simulink model "sampleModel33"  (R2021b)
settings: Solver=VariableStepAuto  StartTime=0.0  StopTime=10.0  RelTol=1e-3
undefined symbols (not defined in the file or in its folder): DiscIntNeverNeededParam, Newton, Raphson
libraries: simulink x17, slpidlib x2
settings Model: Creator=user  LastModifiedBy=user

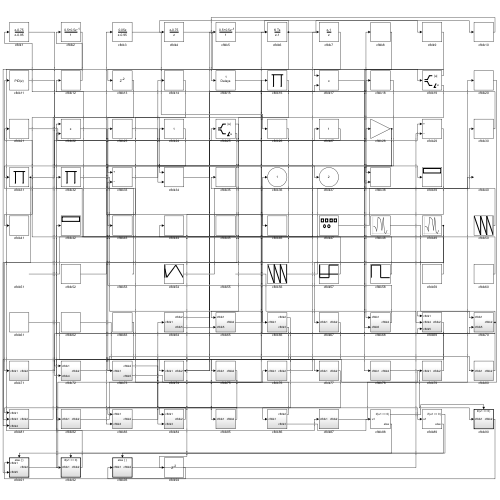
[thumbnail: Simulink's stored preview of the top-level diagram]
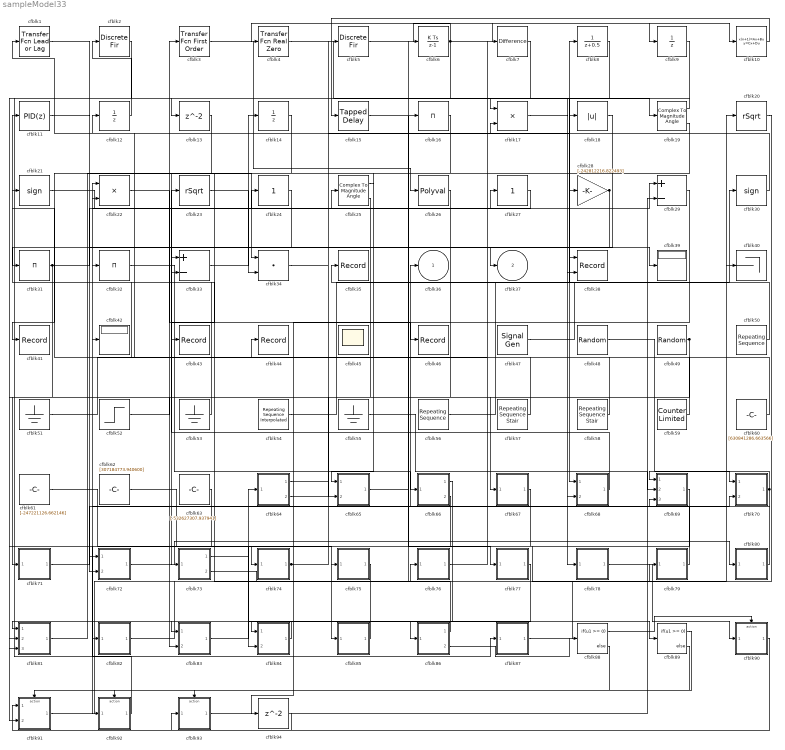
== system sampleModel33 ==
  cfblk1 : simulink/Discrete/Transfer Fcn Lead or Lag  PoleZ=0.95  ZeroZ=0.75  ICPrevOutput=0.0  ICPrevInput=0.0  DoSatur=off
      settings: SourceProductBaseCode=SL
  cfblk10 : DiscreteStateSpace
  cfblk11 : slpidlib/PID Controller  Controller=PID  Form=Parallel  TimeDomain=Discrete-time  UseExternalTs=off  SampleTime=1  IntegratorMethod=Forward Euler  FilterMethod=Forward Euler  ControllerParametersSource=internal  P=1  I=1  D=0  UseFilter=on  N=100  TunerSelectOption=Transfer Function Based (PID Tuner App)  InitialConditionSource=internal  InitialConditionForIntegrator=0  InitialConditionForFilter=0  DifferentiatorICPrevScaledInput=0  ExternalReset=none  TrackingMode=off  Kt=1  LimitOutput=off  SatLimitsSource=internal  UpperSaturationLimit=inf  LowerSaturationLimit=-inf  LinearizeAsGain=off  AntiWindupMode=none  Kb=1  POutMin=[]  POutMax=[]  IOutMin=[]  IOutMax=[]  DOutMin=[]  DOutMax=[]  NOutMin=[]  NOutMax=[]  SumOutMin=[]  SumOutMax=[]  SaturationOutMin=[]  SaturationOutMax=[]  PParamMin=[]  PParamMax=[]  IParamMin=[]  IParamMax=[]  DParamMin=[]  DParamMax=[]  NParamMin=[]  NParamMax=[]  KbParamMin=[]  KbParamMax=[]  KtParamMin=[]  KtParamMax=[]  KbOutMin=[]  KbOutMax=[]  KtOutMin=[]  KtOutMax=[]  IntegratorOutMin=[]  IntegratorOutMax=[]  FilterOutMin=[]  FilterOutMax=[]  SumI1OutMin=[]  SumI1OutMax=[]  SumI2OutMin=[]  SumI2OutMax=[]  SumI3OutMin=[]  SumI3OutMax=[]  SumI4OutMin=[]  SumI4OutMax=[]  SumDOutMin=[]  SumDOutMax=[]  DifferentiatorOutMin=[]  DifferentiatorOutMax=[]  FilterDiffOutCoefMin=[]  FilterDiffOutCoefMax=[]  ReciprocalOutMin=[]  ReciprocalOutMax=[]  SumDenOutMin=[]  SumDenOutMax=[]  SumNumOutMin=[]  SumNumOutMax=[]  DivideOutMin=[]  DivideOutMax=[]  UdiffTsProdOutMin=[]  UdiffTsProdOutMax=[]  NTsProdOutMin=[]  NTsProdOutMax=[]  UintegralTsProdOutMin=[]  UintegralTsProdOutMax=[]  UngainTsProdOutMin=[]  UngainTsProdOutMax=[]  IntegratorContinuousStateAttributes=''  IntegratorStateMustResolveToSignalObject=off  IntegratorRTWStateStorageClass=Auto  FilterContinuousStateAttributes=''  FilterStateMustResolveToSignalObject=off  FilterRTWStateStorageClass=Auto  ParallelPVariant=InternalParameters  IdealPVariant=Disabled  IVariant=InternalParameters  DVariant=InternalParameters  IntegratorVariant=Discrete  SatVariant=Disabled  AWVariant=Passthrough  PCopyVariant=Disabled  TRVariant=Disabled  FdbkBlocksVariant=Forward  IdealPFdbkVariant=Disabled  SatFdbkVariant=Disabled  DerivativeFilterVariant=ForwardEulerFilter  NVariant=InternalParameters  NCopyVariant=Disabled  FilterICVariant=InternalICsFilter  IntegratorICVariant=InternalICs  ExternalResetVariant=Disabled  TRSumVariant=Passthrough  SumFdbkVariant=Disabled  SumVariant=Sum_PID  TsampFilterVariant=InternalTs  TsampNgainVariant=Passthrough  TsampIntegralVariant=Passthrough  ExternalSaturationOutDataTypeStr=Inherit: Same as second input
  cfblk12 : UnitDelay  HasFrameUpgradeWarning=on
  cfblk13 : Delay  SampleTime=1
  cfblk14 : UnitDelay  HasFrameUpgradeWarning=on
  cfblk15 : simulink/Discrete/Tapped Delay  vinit=0.0  samptime=-1  NumDelays=1  DelayOrder=Oldest  includeCurrent=off
  cfblk16 : Product  Inputs=*
  cfblk17 : Product
  cfblk18 : Abs
  cfblk19 : ComplexToMagnitudeAngle
  cfblk2 : DiscreteFir  SampleTime=1
  cfblk20 : Sqrt  Operator=rSqrt  AlgorithmType=Newton-Raphson  SaturateOnIntegerOverflow=on
  cfblk21 : Signum
  cfblk22 : Product
  cfblk23 : Sqrt  Operator=rSqrt  AlgorithmType=Newton-Raphson  SaturateOnIntegerOverflow=on
  cfblk24 : simulink/Math Operations/Slider Gain  gain=1  low=0  high=2
  cfblk25 : ComplexToMagnitudeAngle
  cfblk26 : Polyval  Coefs=[ +2.081618890e-019, -1.441693666e-014, +4.719686976e-010, -8.536869453e-006, +1.621573104e-001, -8.087801117e+001 ]
  cfblk27 : simulink/Math Operations/Slider Gain  gain=1  low=0  high=2
  cfblk28 : Gain  Gain=[-242812216.822493]
  cfblk29 : Sum  Inputs=+-
  cfblk3 : simulink/Discrete/Transfer Fcn First Order  PoleZ=0.95  ICPrevOutput=0.0  DoSatur=off
  cfblk30 : Signum
  cfblk31 : Product  Inputs=*
  cfblk32 : Product  Inputs=*
  cfblk33 : Sum  Inputs=+-
  cfblk34 : DotProduct  InputSameDT=on  OutDataTypeStr=Inherit: Inherit via internal rule
  cfblk35 : Record  FileSettingsInternal="{\"entries\":[{\"content\":{\"excelSettings\":{\"content\":{},\"type\":\"Streamout.ExcelSettings\"}},\"type\":\"Streamout.FileSettingStorage\",\"uuid\":\"35001ed6-113c-4df0-b2ca-dfb1ae9641fd\"}],\"packageUris\":[\"http://schema.mathworks.com/mf0/streamout_blocks/R2020a\"],\"version\":\"1.0\"}"  SignalsInternal="{\"entries\":[{\"content\":{\"signals\":[{\"content\":{\"blockPath\":[\"sampleModel33/cfblk35\"],\"channel\":[],\"dimensions\":[1],\"domain\":\"sampleModel33/cfblk35\",\"lineColor\":\"#7e2f8e\",\"plots\":[1],\"port\":1,\"sid\":[\"\"],\"signalID\":1315,\"signalName\":\"cfblk50\"},\"type\":\"RecordBlkView.Signal\",\"uuid\":\"b51956be-35d7-410c-a634-2c74a70fc2db\"}]},\"type\":\"RecordBlkView.InputSignals\",\"uuid\":\"6f3c5769-0a70-4b4d-8f9e-08021210cbdc\"}],\"packageUris\":[\"http://schema.mathworks.com/mf0/streamout_blocks/R2020a\"],\"version\":\"1.0\"}"  VisualizationBindings="{\"sparklinesplugin\":{\"info\":[{\"bindingParametersList\":[],\"subplotID\":1}]}}"
  cfblk38 : Record  FileSettingsInternal="{\"entries\":[{\"content\":{\"excelSettings\":{\"content\":{},\"type\":\"Streamout.ExcelSettings\"}},\"type\":\"Streamout.FileSettingStorage\",\"uuid\":\"0be8a96a-0af5-42bf-ad20-4a59eb5ad2b5\"}],\"packageUris\":[\"http://schema.mathworks.com/mf0/streamout_blocks/R2020a\"],\"version\":\"1.0\"}"  Layout=[1 1]  SignalsInternal="{\"entries\":[{\"content\":{\"signals\":[{\"content\":{\"blockPath\":[\"sampleModel33/cfblk38\"],\"channel\":[],\"dimensions\":[1],\"domain\":\"sampleModel33/cfblk38\",\"lineColor\":\"#a2142f\",\"plots\":[1],\"port\":1,\"sid\":[\"\"],\"signalID\":1291,\"signalName\":\"cfblk18\"},\"type\":\"RecordBlkView.Signal\",\"uuid\":\"6335e883-a2f0-4c07-b781-486b19723835\"},{\"content\":{\"blockPath\":[\"sampleModel33/cfblk38\"],\"channel\":[],\"dimensions\":[1],\"domain\":\"sampleModel33/cfblk38\",\"lineColor\":\"#139fff\",\"plots\":[1],\"port\":2,\"sid\":[\"\"],\"signalID\":1295,\"signalName\":\"cfblk28\"},\"type\":\"RecordBlkView.Signal\",\"uuid\":\"6659cc2e-0a72-45a6-80d2-b962cd38ef36\"}]},\"type\":\"RecordBlkView.InputSignals\",\"uuid\":\"964d8c4e-428f-4cc5-8505-fdd76ce85f40\"}],\"packageUris\":[\"http://schema.mathworks.com/mf0/streamout_blocks/R2020a\"],\"version\":\"1.0\"}"  VisualizationBindings="{\"xyplotplugin\":{\"info\":[{\"series\":[{\"bindingParametersList\":[{\"parameter\":\"X-Axis\",\"signalID\":1291,\"signalName\":\"cfblk18\"},{\"parameter\":\"Y-Axis\",\"signalID\":1295,\"signalName\":\"cfblk28\"}],\"seriesID\":40894}],\"subplotID\":1}]}}"  CompatibilityTag=XY
  cfblk39 : Display
  cfblk4 : simulink/Discrete/Transfer Fcn Real Zero  ZeroZ=0.75  ICPrevInput=0.0  DoSatur=off
      settings: SourceProductBaseCode=SL
  cfblk40 : Terminator
  cfblk41 : Record  FileSettingsInternal="{\"entries\":[{\"content\":{\"excelSettings\":{\"content\":{},\"type\":\"Streamout.ExcelSettings\"}},\"type\":\"Streamout.FileSettingStorage\",\"uuid\":\"943cf604-ea0c-4e86-a751-38b2b14ebefe\"}],\"packageUris\":[\"http://schema.mathworks.com/mf0/streamout_blocks/R2020a\"],\"version\":\"1.0\"}"  SignalsInternal="{\"entries\":[{\"content\":{\"signals\":[{\"content\":{\"blockPath\":[\"sampleModel33/cfblk41\"],\"channel\":[],\"dimensions\":[1],\"domain\":\"sampleModel33/cfblk41\",\"lineColor\":\"#22b573\",\"plots\":[1],\"port\":1,\"sid\":[\"\"],\"signalID\":1299,\"signalName\":\"cfblk14\"},\"type\":\"RecordBlkView.Signal\",\"uuid\":\"e871c3d6-6255-463e-9a74-0a0ab0dc3673\"}]},\"type\":\"RecordBlkView.InputSignals\",\"uuid\":\"e3ee7eed-40cd-48d9-8ee8-8000d3adafc3\"}],\"packageUris\":[\"http://schema.mathworks.com/mf0/streamout_blocks/R2020a\"],\"version\":\"1.0\"}"  VisualizationBindings="{\"sparklinesplugin\":{\"info\":[{\"bindingParametersList\":[],\"subplotID\":1}]}}"
  cfblk42 : Display
  cfblk43 : Record  FileSettingsInternal="{\"entries\":[{\"content\":{\"excelSettings\":{\"content\":{},\"type\":\"Streamout.ExcelSettings\"}},\"type\":\"Streamout.FileSettingStorage\",\"uuid\":\"3f9b25bd-badb-4d41-b468-b463b58841fb\"}],\"packageUris\":[\"http://schema.mathworks.com/mf0/streamout_blocks/R2020a\"],\"version\":\"1.0\"}"  SignalsInternal="{\"entries\":[{\"content\":{\"signals\":[{\"content\":{\"blockPath\":[\"sampleModel33/cfblk43\"],\"channel\":[],\"dimensions\":[1],\"domain\":\"sampleModel33/cfblk43\",\"lineColor\":\"#0072bd\",\"plots\":[1],\"port\":1,\"sid\":[\"\"],\"signalID\":1303,\"signalName\":\"cfblk19:2\"},\"type\":\"RecordBlkView.Signal\",\"uuid\":\"9792fccf-e420-4e25-ab06-4eadf706866a\"}]},\"type\":\"RecordBlkView.InputSignals\",\"uuid\":\"96c16f90-f0aa-40b6-afa4-1459bd73ce77\"}],\"packageUris\":[\"http://schema.mathworks.com/mf0/streamout_blocks/R2020a\"],\"version\":\"1.0\"}"  VisualizationBindings="{\"sparklinesplugin\":{\"info\":[{\"bindingParametersList\":[],\"subplotID\":1}]}}"
  cfblk44 : Record  FileSettingsInternal="{\"entries\":[{\"content\":{\"excelSettings\":{\"content\":{},\"type\":\"Streamout.ExcelSettings\"}},\"type\":\"Streamout.FileSettingStorage\",\"uuid\":\"f2588ed7-79e1-4caa-a079-da7ab20d12fc\"}],\"packageUris\":[\"http://schema.mathworks.com/mf0/streamout_blocks/R2020a\"],\"version\":\"1.0\"}"  SignalsInternal="{\"entries\":[{\"content\":{\"signals\":[{\"content\":{\"blockPath\":[\"sampleModel33/cfblk44\"],\"channel\":[],\"dimensions\":[1],\"domain\":\"sampleModel33/cfblk44\",\"lineColor\":\"#77ac30\",\"plots\":[1],\"port\":1,\"sid\":[\"\"],\"signalID\":1319,\"signalName\":\"cfblk58\"},\"type\":\"RecordBlkView.Signal\",\"uuid\":\"acc73365-e21f-4d8b-96ab-155052806760\"}]},\"type\":\"RecordBlkView.InputSignals\",\"uuid\":\"d7a8ec08-6dc6-46d4-b733-eb162bbe280f\"}],\"packageUris\":[\"http://schema.mathworks.com/mf0/streamout_blocks/R2020a\"],\"version\":\"1.0\"}"  VisualizationBindings="{\"sparklinesplugin\":{\"info\":[{\"bindingParametersList\":[],\"subplotID\":1}]}}"
  cfblk45 : Scope
      settings: Floating=on
  cfblk46 : Record  FileSettingsInternal="{\"entries\":[{\"content\":{\"excelSettings\":{\"content\":{},\"type\":\"Streamout.ExcelSettings\"}},\"type\":\"Streamout.FileSettingStorage\",\"uuid\":\"2d09eccc-ab10-47b1-af95-cecebc9448e0\"}],\"packageUris\":[\"http://schema.mathworks.com/mf0/streamout_blocks/R2020a\"],\"version\":\"1.0\"}"  SignalsInternal="{\"entries\":[{\"content\":{\"signals\":[{\"content\":{\"blockPath\":[\"sampleModel33/cfblk46\"],\"channel\":[],\"dimensions\":[1],\"domain\":\"sampleModel33/cfblk46\",\"lineColor\":\"#d95319\",\"plots\":[1],\"port\":1,\"sid\":[\"\"],\"signalID\":1307,\"signalName\":\"cfblk22\"},\"type\":\"RecordBlkView.Signal\",\"uuid\":\"5f2a2cab-08a1-4387-b816-50fa2120540d\"}]},\"type\":\"RecordBlkView.InputSignals\",\"uuid\":\"c9b5cd79-e6b9-468f-9bb4-0740aaf235d3\"}],\"packageUris\":[\"http://schema.mathworks.com/mf0/streamout_blocks/R2020a\"],\"version\":\"1.0\"}"  VisualizationBindings="{\"sparklinesplugin\":{\"info\":[{\"bindingParametersList\":[],\"subplotID\":1}]}}"
  cfblk47 : SignalGenerator  WaveForm=sawtooth  Amplitude=[-806395238.078433]
  cfblk48 : RandomNumber  Mean=[46041.065691]  Variance=[79471.340689]  Seed=[573569622.000000]  SampleTime=0.1
  cfblk49 : RandomNumber  Mean=[-27661.970417]  Variance=[16133.365811]  Seed=[886370585.000000]  SampleTime=0.1
  cfblk5 : DiscreteFir  SampleTime=1
  cfblk50 : simulink/Sources/Repeating Sequence  rep_seq_t=[0 2]  rep_seq_y=[803997380.811525, 517164280.997497]
  cfblk51 : Ground
  cfblk52 : Step  Time=[18.000000]  Before=[-7550237.569274]  After=[317370971.728037]  SampleTime=0
  cfblk53 : Ground
  cfblk54 : simulink/Sources/Repeating Sequence Interpolated  OutValues=[-422066434.065173, -713885697.695092, -383733753.736717, -305117400.776015, -720923073.966345]  TimeValues=[0 0.1 0.5 0.6 1].'  LookUpMeth=Interpolation-Use End Values  tsamp=0.01  OutMin=[]  OutMax=[]  OutDataTypeStr=double  OutputDataTypeScalingMode=double  OutDataType=fixdt(0,8)  OutScaling=2^-10
  cfblk55 : Ground
  cfblk56 : simulink/Sources/Repeating Sequence  rep_seq_t=[0 2]  rep_seq_y=[111643374.462294, -897632520.777855]
  cfblk57 : simulink/Sources/Repeating Sequence Stair  OutValues=[-165294741.865797, 423160325.966491]  tsamp=-1  OutMin=[]  OutMax=[]  OutDataTypeStr=double  OutputDataTypeScalingMode=double  OutDataType=fixdt(0,8)  ConRadixGroup=Best Precision: Vector-wise  OutScaling=2^-12
  cfblk58 : simulink/Sources/Repeating Sequence Stair  OutValues=[758546070.290987, 202958879.064606]  tsamp=-1  OutMin=[]  OutMax=[]  OutDataTypeStr=double  OutputDataTypeScalingMode=double  OutDataType=fixdt(0,8)  ConRadixGroup=Best Precision: Vector-wise  OutScaling=2^-12
  cfblk59 : simulink/Sources/Counter Limited  uplimit=[465.000000]  tsamp=-1
  cfblk6 : DiscreteIntegrator  ICPrevOutput=DiscIntNeverNeededParam  ICPrevScaledInput=DiscIntNeverNeededParam
  cfblk60 : Constant  Value=[630841286.663566]  SampleTime=1
  cfblk61 : Constant  Value=[-247221126.662146]  SampleTime=1
  cfblk62 : Constant  Value=[307184773.940600]  SampleTime=1
  cfblk63 : Constant  Value=[-532627307.937941]  SampleTime=1
  cfblk64 : Subsystem
  cfblk65 : Subsystem
  cfblk66 : Subsystem
  cfblk67 : Subsystem
  cfblk68 : Subsystem
  cfblk69 : Subsystem
  cfblk7 : simulink/Discrete/Difference  ICPrevInput=0.0  OutMin=[]  OutMax=[]  OutDataTypeStr=Inherit: Inherit via back propagation  OutDataType=fixdt(1, 16)  OutScaling=2^-10  DoSatur=off
  cfblk70 : Subsystem
  cfblk71 : Subsystem
  cfblk72 : Subsystem
  cfblk73 : Subsystem
  cfblk74 : Subsystem
  cfblk75 : Subsystem
  cfblk76 : Subsystem
  cfblk77 : Subsystem
  cfblk78 : Subsystem
  cfblk79 : Subsystem
  cfblk8 : DiscreteTransferFcn  SampleTime=1
  cfblk80 : Subsystem
  cfblk81 : Subsystem
  cfblk82 : Subsystem
  cfblk83 : Subsystem
  cfblk84 : Subsystem
  cfblk85 : Subsystem
  cfblk86 : Subsystem
  cfblk87 : Subsystem
  cfblk88 : If  IfExpression=u1 >= 0  SampleTime=1
  cfblk89 : If  IfExpression=u1 >= 0  SampleTime=1
  cfblk9 : UnitDelay  HasFrameUpgradeWarning=on
  cfblk90 : Subsystem  TreatAsAtomicUnit=on
  cfblk91 : Subsystem  TreatAsAtomicUnit=on
  cfblk92 : Subsystem  TreatAsAtomicUnit=on
  cfblk93 : Subsystem  TreatAsAtomicUnit=on
  cfblk94 : Delay  SampleTime=1
  cfblk36 : Outport
  cfblk37 : Outport  Port=2
  wires:
  cfblk80/1(cfblk2) -> cfblk22/1
  cfblk77/1(cfblk2) -> cfblk86/1(cfblk1)
  cfblk20/1 -> cfblk74/1(cfblk1)
  cfblk78/1(cfblk2) -> cfblk90/1(cfblk1)
  cfblk72/1(cfblk2) -> cfblk80/1(cfblk1)
  cfblk81/1(cfblk2) -> cfblk34/1
  cfblk2/1 -> cfblk87/1(cfblk1)
  cfblk48/1 -> cfblk70/1(cfblk1)
  cfblk92/1(cfblk2) -> cfblk42/1
  cfblk91/1(cfblk2) -> cfblk79/1(cfblk1)
  cfblk21/1 -> cfblk24/1
  cfblk27/1 -> cfblk22/2
  cfblk23/1 -> cfblk39/1
  cfblk62/1 -> cfblk85/1(cfblk1)
  cfblk13/1 -> cfblk73/1(cfblk1)
  cfblk5/1 -> cfblk9/1
  cfblk58/1 -> cfblk44/1
  cfblk3/1 -> cfblk26/1
  cfblk53/1 -> cfblk11/1
  cfblk69/1(cfblk2) -> cfblk75/1(cfblk1)
  cfblk73/1(cfblk2) -> cfblk89/1
  cfblk28/1 -> cfblk31/1, cfblk38/2
  cfblk56/1 -> cfblk8/1
  cfblk10/1 -> cfblk15/1
  cfblk49/1 -> cfblk71/1(cfblk1), cfblk67/1(cfblk1)
  cfblk9/1 -> cfblk68/1(cfblk1)
  cfblk59/1 -> cfblk32/1
  cfblk85/1(cfblk2) -> cfblk81/1(cfblk1)
  cfblk31/1 -> cfblk25/1, cfblk81/3(cfblk4)
  cfblk65/1(cfblk2) -> cfblk6/1
  cfblk82/1(cfblk2) -> cfblk16/1
  cfblk47/1 -> cfblk30/1
  cfblk7/1 -> cfblk13/1
  cfblk73/2(cfblk5) -> cfblk76/1(cfblk1)
  cfblk79/1(cfblk2) -> cfblk36/1
  cfblk16/1 -> cfblk65/1(cfblk1)
  cfblk12/1 -> cfblk2/1
  cfblk68/1(cfblk2) -> cfblk23/1
  cfblk15/1 -> cfblk77/1(cfblk1)
  cfblk17/1 -> cfblk78/1(cfblk1)
  cfblk8/1 -> cfblk68/2(cfblk5)
  cfblk76/1(cfblk2) -> cfblk29/1
  cfblk87/1(cfblk2) -> cfblk40/1
  cfblk57/1 -> cfblk21/1
  cfblk33/1 -> cfblk14/1
  cfblk66/1(cfblk2) -> cfblk84/1(cfblk1)
  cfblk52/1 -> cfblk3/1
  cfblk32/1 -> cfblk66/1(cfblk1)
  cfblk60/1 -> cfblk12/1
  cfblk90/1(cfblk2) -> cfblk91/1(cfblk1)
  cfblk75/1(cfblk2) -> cfblk92/1(cfblk1)
  cfblk83/1(cfblk2) -> cfblk64/1(cfblk1)
  cfblk67/1(cfblk2) -> cfblk82/1(cfblk1)
  cfblk6/1 -> cfblk10/1, cfblk4/1, cfblk91/2(cfblk5)
  cfblk11/1 -> cfblk37/1
  cfblk25/1 -> cfblk34/2
  cfblk93/1(cfblk2) -> cfblk29/2
  cfblk84/1(cfblk2) -> cfblk83/1(cfblk1)
  cfblk4/1 -> cfblk19/1
  cfblk63/1 -> cfblk81/2(cfblk3)
  cfblk22/1 -> cfblk46/1
  cfblk14/1 -> cfblk41/1
  cfblk24/1 -> cfblk33/1
  cfblk74/1(cfblk2) -> cfblk27/1, cfblk17/2
  cfblk26/1 -> cfblk83/2(cfblk3)
  cfblk64/1(cfblk2) -> cfblk28/1
  cfblk1/1 -> cfblk72/1(cfblk1)
  cfblk19/1 -> cfblk17/1
  cfblk71/1(cfblk2) -> cfblk70/2(cfblk5)
  cfblk64/2(cfblk5) -> cfblk18/1
  cfblk34/1 -> cfblk5/1
  cfblk61/1 -> cfblk84/2(cfblk3)
  cfblk70/1(cfblk2) -> cfblk69/1(cfblk1), cfblk69/3(cfblk5)
  cfblk54/1 -> cfblk20/1
  cfblk86/1(cfblk2) -> cfblk33/2
  cfblk66/2(cfblk3) -> cfblk72/2(cfblk4)
  cfblk55/1 -> cfblk69/2(cfblk4)
  cfblk18/1 -> cfblk38/1
  cfblk51/1 -> cfblk7/1
  cfblk30/1 -> cfblk1/1
  cfblk86/2(cfblk3) -> cfblk88/1
  cfblk19/2 -> cfblk43/1
  cfblk25/2 -> cfblk65/2(cfblk5)
  cfblk50/1 -> cfblk35/1
  cfblk88/1 -> cfblk90/Action
  cfblk88/2 -> cfblk91/Action
  cfblk89/1 -> cfblk92/Action
  cfblk89/2 -> cfblk93/Action
  cfblk29/1 -> cfblk94/1
  cfblk94/1 -> cfblk93/1(cfblk1)

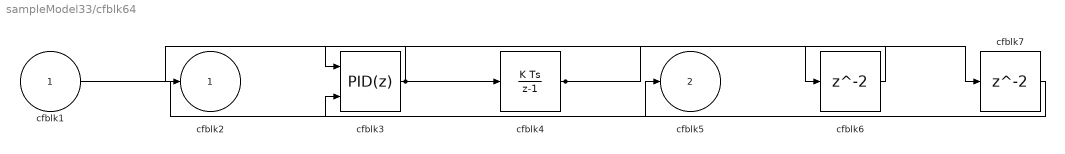
== system sampleModel33/cfblk64 ==
  cfblk1 : Inport
  cfblk3 : slpidlib/PID Controller (2DOF)  Controller=PID  Form=Parallel  TimeDomain=Discrete-time  UseExternalTs=off  SampleTime=1  IntegratorMethod=Forward Euler  FilterMethod=Forward Euler  ControllerParametersSource=internal  P=1  I=1  D=0  UseFilter=on  N=100  b=1  c=1  TunerSelectOption=Transfer Function Based (PID Tuner App)  InitialConditionSource=internal  InitialConditionForIntegrator=0  InitialConditionForFilter=0  DifferentiatorICPrevScaledInput=0  ExternalReset=none  TrackingMode=off  Kt=1  LimitOutput=off  SatLimitsSource=internal  UpperSaturationLimit=inf  LowerSaturationLimit=-inf  LinearizeAsGain=off  AntiWindupMode=none  Kb=1  POutMin=[]  POutMax=[]  IOutMin=[]  IOutMax=[]  DOutMin=[]  DOutMax=[]  NOutMin=[]  NOutMax=[]  bOutMin=[]  bOutMax=[]  cOutMin=[]  cOutMax=[]  SumOutMin=[]  SumOutMax=[]  SaturationOutMin=[]  SaturationOutMax=[]  PParamMin=[]  PParamMax=[]  IParamMin=[]  IParamMax=[]  DParamMin=[]  DParamMax=[]  NParamMin=[]  NParamMax=[]  bParamMin=[]  bParamMax=[]  cParamMin=[]  cParamMax=[]  KbParamMin=[]  KbParamMax=[]  KtParamMin=[]  KtParamMax=[]  KbOutMin=[]  KbOutMax=[]  KtOutMin=[]  KtOutMax=[]  IntegratorOutMin=[]  IntegratorOutMax=[]  FilterOutMin=[]  FilterOutMax=[]  SumI1OutMin=[]  SumI1OutMax=[]  SumI2OutMin=[]  SumI2OutMax=[]  SumI3OutMin=[]  SumI3OutMax=[]  SumI4OutMin=[]  SumI4OutMax=[]  SumDOutMin=[]  SumDOutMax=[]  Sum1OutMin=[]  Sum1OutMax=[]  Sum2OutMin=[]  Sum2OutMax=[]  Sum3OutMin=[]  Sum3OutMax=[]  DifferentiatorOutMin=[]  DifferentiatorOutMax=[]  FilterDiffOutCoefMin=[]  FilterDiffOutCoefMax=[]  ReciprocalOutMin=[]  ReciprocalOutMax=[]  SumDenOutMin=[]  SumDenOutMax=[]  SumNumOutMin=[]  SumNumOutMax=[]  DivideOutMin=[]  DivideOutMax=[]  UdiffTsProdOutMin=[]  UdiffTsProdOutMax=[]  NTsProdOutMin=[]  NTsProdOutMax=[]  UintegralTsProdOutMin=[]  UintegralTsProdOutMax=[]  UngainTsProdOutMin=[]  UngainTsProdOutMax=[]  IntegratorContinuousStateAttributes=''  IntegratorStateMustResolveToSignalObject=off  IntegratorRTWStateStorageClass=Auto  FilterContinuousStateAttributes=''  FilterStateMustResolveToSignalObject=off  FilterRTWStateStorageClass=Auto  ParallelPVariant=InternalParameters  IdealPVariant=Disabled  IVariant=InternalParameters  DVariant=InternalParameters  bVariant=InternalParameters  cVariant=InternalParameters  IntegratorVariant=Discrete  SatVariant=Disabled  AWVariant=Passthrough  PCopyVariant=Disabled  TRVariant=Disabled  FdbkBlocksVariant=Forward  IdealPFdbkVariant=Disabled  SatFdbkVariant=Disabled  DerivativeFilterVariant=ForwardEulerFilter  NVariant=InternalParameters  NCopyVariant=Disabled  FilterICVariant=InternalICsFilter  IntegratorICVariant=InternalICs  ExternalResetVariant=Disabled  TRSumVariant=Passthrough  SumFdbkVariant=Disabled  SumVariant=Sum_PID  TsampFilterVariant=InternalTs  TsampNgainVariant=Passthrough  TsampIntegralVariant=Passthrough  ExternalSaturationOutDataTypeStr=Inherit: Same as second input
      settings: SourceProductBaseCode=SL
  cfblk4 : DiscreteIntegrator  ICPrevOutput=DiscIntNeverNeededParam  ICPrevScaledInput=DiscIntNeverNeededParam
  cfblk6 : Delay  SampleTime=1
  cfblk7 : Delay  SampleTime=1
  cfblk2 : Outport
  cfblk5 : Outport  Port=2
  wires:
  cfblk4/1 -> cfblk6/1, cfblk7/1
  cfblk3/1 -> cfblk4/1, cfblk2/1
  cfblk1/1 -> cfblk5/1
  cfblk6/1 -> cfblk3/1
  cfblk7/1 -> cfblk3/2

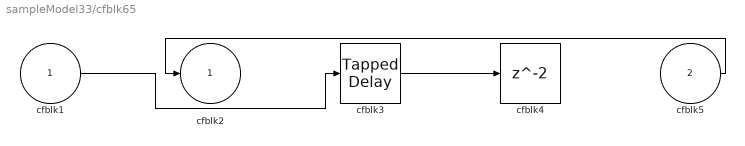
== system sampleModel33/cfblk65 ==
  cfblk1 : Inport
  cfblk5 : Inport  Port=2
  cfblk3 : simulink/Discrete/Tapped Delay  vinit=0.0  samptime=-1  NumDelays=1  DelayOrder=Oldest  includeCurrent=off
  cfblk4 : Delay  SampleTime=1
  cfblk2 : Outport
  wires:
  cfblk5/1 -> cfblk2/1
  cfblk1/1 -> cfblk3/1
  cfblk3/1 -> cfblk4/1

== system sampleModel33/cfblk66 ==
  cfblk1 : Inport
  cfblk2 : Outport
  cfblk3 : Outport  Port=2
  wires:
  cfblk1/1 -> cfblk2/1, cfblk3/1

== system sampleModel33/cfblk67 ==
  cfblk1 : Inport
  cfblk3 : Constant  Value=[-570837548.710489]  SampleTime=1
  cfblk2 : Outport
  wires:
  cfblk3/1 -> cfblk2/1

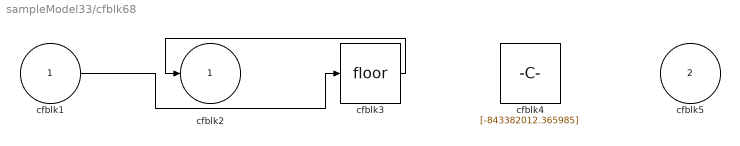
== system sampleModel33/cfblk68 ==
  cfblk1 : Inport
  cfblk5 : Inport  Port=2
  cfblk3 : Rounding
  cfblk4 : Constant  Value=[-843382012.365985]  SampleTime=1
  cfblk2 : Outport
  wires:
  cfblk3/1 -> cfblk2/1
  cfblk1/1 -> cfblk3/1

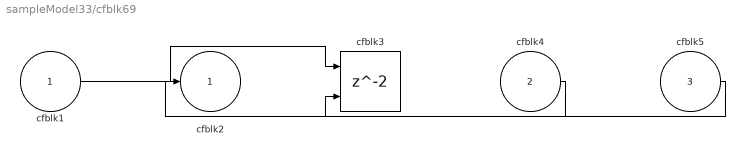
== system sampleModel33/cfblk69 ==
  cfblk1 : Inport
  cfblk4 : Inport  Port=2
  cfblk5 : Inport  Port=3
  cfblk3 : Delay  ShowEnablePort=on  SampleTime=1
      settings: InputPortMap=u0,e6
  cfblk2 : Outport
  wires:
  cfblk1/1 -> cfblk3/1
  cfblk5/1 -> cfblk2/1
  cfblk4/1 -> cfblk3/2

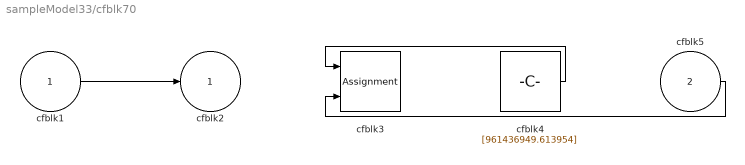
== system sampleModel33/cfblk70 ==
  cfblk1 : Inport
  cfblk5 : Inport  Port=2
  cfblk3 : Assignment  DiagnosticForDimensions=Warning  IndexOptions=Index vector (dialog)  Indices=1  OutputSizes=1
  cfblk4 : Constant  Value=[961436949.613954]  SampleTime=1
  cfblk2 : Outport
  wires:
  cfblk1/1 -> cfblk2/1
  cfblk4/1 -> cfblk3/1
  cfblk5/1 -> cfblk3/2

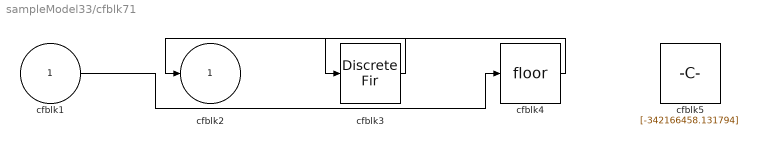
== system sampleModel33/cfblk71 ==
  cfblk1 : Inport
  cfblk3 : DiscreteFir  SampleTime=1
  cfblk4 : Rounding
  cfblk5 : Constant  Value=[-342166458.131794]  SampleTime=1
  cfblk2 : Outport
  wires:
  cfblk3/1 -> cfblk2/1
  cfblk1/1 -> cfblk4/1
  cfblk4/1 -> cfblk3/1

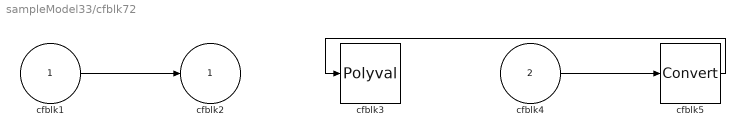
== system sampleModel33/cfblk72 ==
  cfblk1 : Inport
  cfblk4 : Inport  Port=2
  cfblk3 : Polyval  Coefs=[ +2.081618890e-019, -1.441693666e-014, +4.719686976e-010, -8.536869453e-006, +1.621573104e-001, -8.087801117e+001 ]
  cfblk5 : DataTypeConversion
  cfblk2 : Outport
  wires:
  cfblk1/1 -> cfblk2/1
  cfblk4/1 -> cfblk5/1
  cfblk5/1 -> cfblk3/1

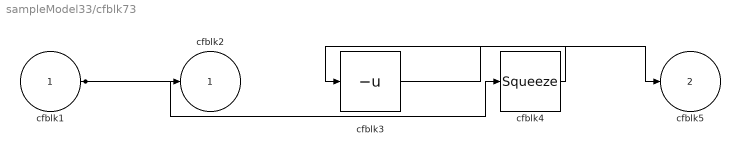
== system sampleModel33/cfblk73 ==
  cfblk1 : Inport
  cfblk3 : UnaryMinus
  cfblk4 : Squeeze
  cfblk2 : Outport
  cfblk5 : Outport  Port=2
  wires:
  cfblk4/1 -> cfblk3/1
  cfblk1/1 -> cfblk4/1, cfblk2/1
  cfblk3/1 -> cfblk5/1

== system sampleModel33/cfblk74 ==
  cfblk1 : Inport
  cfblk3 : Delay  ShowEnablePort=on  SampleTime=1
      settings: InputPortMap=u0,e6
  cfblk2 : Outport
  wires:
  cfblk1/1 -> cfblk3/1, cfblk3/2
  cfblk3/1 -> cfblk2/1

== system sampleModel33/cfblk75 ==
  cfblk1 : Inport
  cfblk3 : simulink/Math Operations/Slider Gain  gain=1  low=0  high=2
  cfblk2 : Outport
  wires:
  cfblk1/1 -> cfblk2/1, cfblk3/1

== system sampleModel33/cfblk76 ==
  cfblk1 : Inport
  cfblk3 : Abs
  cfblk2 : Outport
  wires:
  cfblk1/1 -> cfblk2/1, cfblk3/1

== system sampleModel33/cfblk77 ==
  cfblk1 : Inport
  cfblk3 : DotProduct  InputSameDT=on  OutDataTypeStr=Inherit: Inherit via internal rule
  cfblk2 : Outport
  wires:
  cfblk1/1 -> cfblk3/1, cfblk3/2
  cfblk3/1 -> cfblk2/1

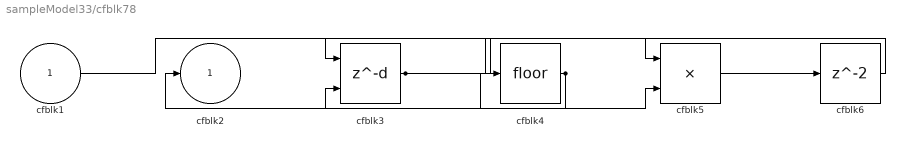
== system sampleModel33/cfblk78 ==
  cfblk1 : Inport
  cfblk3 : Delay  DelayLengthSource=Input port  SampleTime=1
      settings: InputPortMap=u0,p1
  cfblk4 : Rounding
  cfblk5 : Product  Inputs=**
  cfblk6 : Delay  SampleTime=1
  cfblk2 : Outport
  wires:
  cfblk3/1 -> cfblk5/1, cfblk5/2
  cfblk4/1 -> cfblk2/1, cfblk3/2
  cfblk1/1 -> cfblk4/1
  cfblk5/1 -> cfblk6/1
  cfblk6/1 -> cfblk3/1

== system sampleModel33/cfblk79 ==
  cfblk1 : Inport
  cfblk3 : Abs
  cfblk2 : Outport
  wires:
  cfblk1/1 -> cfblk3/1
  cfblk3/1 -> cfblk2/1

== system sampleModel33/cfblk80 ==
  cfblk1 : Inport
  cfblk3 : DiscreteStateSpace
  cfblk4 : simulink/Discrete/Tapped Delay  vinit=0.0  samptime=-1  NumDelays=1  DelayOrder=Oldest  includeCurrent=off
  cfblk5 : Product  Inputs=*
  cfblk2 : Outport
  wires:
  cfblk3/1 -> cfblk2/1
  cfblk5/1 -> cfblk4/1
  cfblk1/1 -> cfblk5/1
  cfblk4/1 -> cfblk3/1

== system sampleModel33/cfblk81 ==
  cfblk1 : Inport
  cfblk3 : Inport  Port=2
  cfblk4 : Inport  Port=3
  cfblk2 : Outport
  wires:
  cfblk1/1 -> cfblk2/1

== system sampleModel33/cfblk82 ==
  cfblk1 : Inport
  cfblk3 : ComplexToMagnitudeAngle
  cfblk4 : Constant  Value=[130734066.386793]  SampleTime=1
  cfblk2 : Outport
  wires:
  cfblk1/1 -> cfblk2/1
  cfblk4/1 -> cfblk3/1

== system sampleModel33/cfblk83 ==
  cfblk1 : Inport
  cfblk3 : Inport  Port=2
  cfblk2 : Outport
  wires:
  cfblk1/1 -> cfblk2/1

== system sampleModel33/cfblk84 ==
  cfblk1 : Inport
  cfblk3 : Inport  Port=2
  cfblk2 : Outport
  wires:
  cfblk1/1 -> cfblk2/1

== system sampleModel33/cfblk85 ==
  cfblk1 : Inport
  cfblk3 : PermuteDimensions
  cfblk2 : Outport
  wires:
  cfblk1/1 -> cfblk3/1
  cfblk3/1 -> cfblk2/1

== system sampleModel33/cfblk86 ==
  cfblk1 : Inport
  cfblk2 : Outport
  cfblk3 : Outport  Port=2
  wires:
  cfblk1/1 -> cfblk3/1, cfblk2/1

== system sampleModel33/cfblk87 ==
  cfblk1 : Inport
  cfblk3 : simulink/Discrete/Tapped Delay  vinit=0.0  samptime=-1  NumDelays=1  DelayOrder=Oldest  includeCurrent=off
  cfblk4 : Rounding
  cfblk2 : Outport
  wires:
  cfblk4/1 -> cfblk2/1
  cfblk1/1 -> cfblk3/1
  cfblk3/1 -> cfblk4/1

== system sampleModel33/cfblk90 ==
  cfblk1 : Inport
  Action Port : ActionPort  ActionPortLabel=if(u1 >= 0)
  cfblk3 : Sum  Inputs=-+
  cfblk2 : Outport
  wires:
  cfblk1/1 -> cfblk3/1, cfblk3/2
  cfblk3/1 -> cfblk2/1

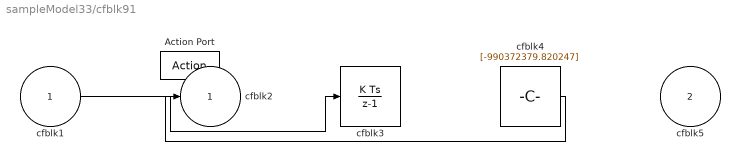
== system sampleModel33/cfblk91 ==
  cfblk1 : Inport
  cfblk5 : Inport  Port=2
  Action Port : ActionPort  ActionPortLabel=else
  cfblk3 : DiscreteIntegrator  SampleTime=-1  ICPrevOutput=DiscIntNeverNeededParam  ICPrevScaledInput=DiscIntNeverNeededParam
  cfblk4 : Constant  Value=[-990372379.820247]  SampleTime=1
  cfblk2 : Outport
  wires:
  cfblk1/1 -> cfblk3/1
  cfblk4/1 -> cfblk2/1

== system sampleModel33/cfblk92 ==
  cfblk1 : Inport
  Action Port : ActionPort  ActionPortLabel=if(u1 >= 0)
  cfblk3 : MinMax  Function=max  Inputs=2
  cfblk2 : Outport
  wires:
  cfblk1/1 -> cfblk2/1, cfblk3/1, cfblk3/2

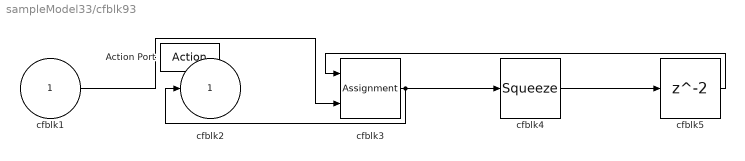
== system sampleModel33/cfblk93 ==
  cfblk1 : Inport
  Action Port : ActionPort  ActionPortLabel=else
  cfblk3 : Assignment  DiagnosticForDimensions=Warning  IndexOptions=Index vector (dialog)  Indices=1  OutputSizes=1
  cfblk4 : Squeeze
  cfblk5 : Delay
  cfblk2 : Outport
  wires:
  cfblk3/1 -> cfblk2/1, cfblk4/1
  cfblk1/1 -> cfblk3/2
  cfblk4/1 -> cfblk5/1
  cfblk5/1 -> cfblk3/1
